simulink model "forward_inverse"  (R2022b)
settings: Solver=VariableStepAuto  StartTime=0.0  StopTime=10.0  RelTol=1e-3
settings Model: Creator=jeffk  LastModifiedBy=jeffk

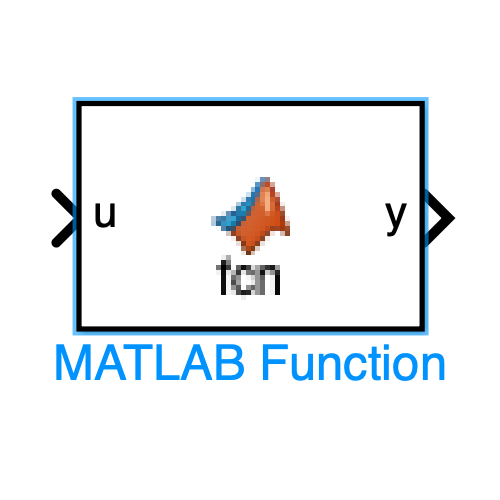
[thumbnail: Simulink's stored preview of the top-level diagram]
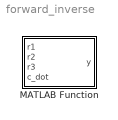
== system forward_inverse ==
  MATLAB Function : MATLAB Function  TreatAsAtomicUnit=on

== matlab function forward_inverse/MATLAB Function ==
  data: r1 input; y output; r2 input; r3 input; c_dot input
function y = fcn(r1, r2, r3, c_dot)
% This will be the forward Jacobian
% the paramaters r are arrays of size three of format: [x, y, theta]
% c_dot is the column vector of the derivative of the cluster variables
% c_dot{1} : x_c
% c_dot{2} : y_c
% c_dot{3} : theta_c
% c_dot{4} : phi_1
% c_dot{5} : phi_2
% c_dot{6} : phi_3
% c_dot{7} : p
% c_dot{8} : q
% c_dot{9} : beta

syms x1 y1 th1 x2 y2 th2 x3 y3 th3

x_c = (x1 + x2 + x3)/3.0;
y_c = (y1 + y2 + y3)/3.0;
theta_c = atan2( (2.0/3.0) * x1 - (1.0/3.0) * (x2 + x3), (2.0/3.0) * y1 - (1.0/3.0) * (y2 + y3));
phi_1 = th1 + theta_c;
phi_2 = th2 + theta_c;
phi_3 = th3 + theta_c;
p = sqrt( (x1 - x2)^2 + (y1 - y2)^2);
q = sqrt( (x3 - x1)^2 + (y3 - y1)^2);
beta = acos( (p^2 + q^2 - (x3 - x2)^2 - (y3 - y2)^2) / (2 * p * q));


F = [x_c, y_c, theta_c, phi_1, phi_2, phi_3, p, q, beta];
X = [x1, y1, th1, x2, y2, th2, x3, y3, th3];

J = jacobian(F, X);
J_inv = inv(J);

J_inv_with_current_values = double( subs (J_inv, [x1, y1, th1, x2, y2, th2, x3, y3, th3], [r1{1}, r1{2}, r1{3}, r2{1}, r2{2}, r2{3}, r3{1}, r3{2}, r3{3}]) );

R_dot = J_inv_with_current_values * [r1{1}; r1{2}; r1{3}; r2{1}; r2{2}; r2{3}; r3{1}; r3{2}; r3{3}];

y = R_dot;
